simulink model "CTRNN"  (Simulink 7.5)
settings: Solver=ode45  StartTime=0.0  StopTime=10.0  MaxStep=0.1  RelTol=1e-3
settings Model: Creator=richard  LastModifiedBy=richard

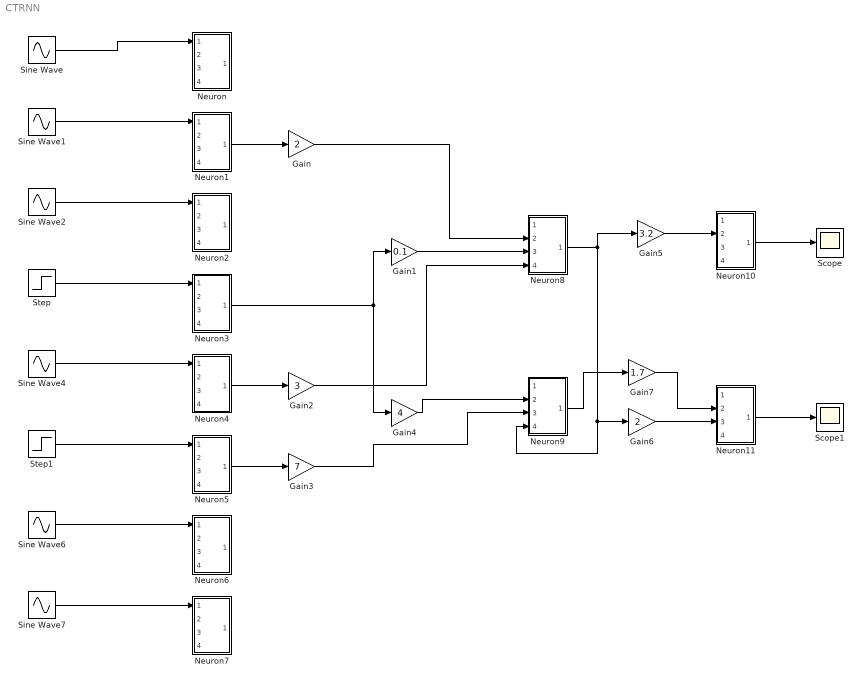
== system CTRNN ==
  Gain : Gain  Gain=2  ParameterDataType=fixdt(1, 16)  ParameterScaling=2^0  OutDataType=fixdt(1, 16)  OutScaling=2^0
  Gain1 : Gain  Gain=0.1  ParameterDataType=fixdt(1, 16)  ParameterScaling=2^0  OutDataType=fixdt(1, 16)  OutScaling=2^0
  Gain2 : Gain  Gain=3  ParameterDataType=fixdt(1, 16)  ParameterScaling=2^0  OutDataType=fixdt(1, 16)  OutScaling=2^0
  Gain3 : Gain  Gain=7  ParameterDataType=fixdt(1, 16)  ParameterScaling=2^0  OutDataType=fixdt(1, 16)  OutScaling=2^0
  Gain4 : Gain  Gain=4  ParameterDataType=fixdt(1, 16)  ParameterScaling=2^0  OutDataType=fixdt(1, 16)  OutScaling=2^0
  Gain5 : Gain  Gain=3.2  ParameterDataType=fixdt(1, 16)  ParameterScaling=2^0  OutDataType=fixdt(1, 16)  OutScaling=2^0
  Gain6 : Gain  Gain=2  ParameterDataType=fixdt(1, 16)  ParameterScaling=2^0  OutDataType=fixdt(1, 16)  OutScaling=2^0
  Gain7 : Gain  Gain=1.7  ParameterDataType=fixdt(1, 16)  ParameterScaling=2^0  OutDataType=fixdt(1, 16)  OutScaling=2^0
  Neuron : Subsystem
  Neuron1 : Subsystem
  Neuron10 : Subsystem
  Neuron11 : Subsystem
  Neuron2 : Subsystem
  Neuron3 : Subsystem
  Neuron4 : Subsystem
  Neuron5 : Subsystem
  Neuron6 : Subsystem
  Neuron7 : Subsystem
  Neuron8 : Subsystem
  Neuron9 : Subsystem
  Scope : Scope
  Scope1 : Scope
  Sine Wave{,1..2,4,6..7} (6 alike) : Sin  Amplitude=1  Bias=0  Frequency=1  Phase=0  Samples=10  SampleTime=0  Offset=0
  Step : Step  SampleTime=0
  Step1 : Step  Time=4  SampleTime=0
  wires:
  Sine Wave7/1 -> Neuron7/1(In1)
  Sine Wave6/1 -> Neuron6/1(In1)
  Step1/1 -> Neuron5/1(In1)
  Sine Wave4/1 -> Neuron4/1(In1)
  Step/1 -> Neuron3/1(In1)
  Sine Wave2/1 -> Neuron2/1(In1)
  Sine Wave1/1 -> Neuron1/1(In1)
  Sine Wave/1 -> Neuron/1(In1)
  Neuron1/1(Out1) -> Gain/1
  Neuron3/1(Out1) -> Gain1/1, Gain4/1
  Neuron4/1(Out1) -> Gain2/1
  Neuron8/1(Out1) -> Neuron9/4(In4), Gain6/1, Gain5/1
  Neuron9/1(Out1) -> Gain7/1
  Neuron10/1(Out1) -> Scope/1
  Neuron11/1(Out1) -> Scope1/1
  Neuron5/1(Out1) -> Gain3/1
  Gain/1 -> Neuron8/2(In2)
  Gain2/1 -> Neuron8/4(In4)
  Gain3/1 -> Neuron9/3(In3)
  Gain1/1 -> Neuron8/3(In3)
  Gain4/1 -> Neuron9/2(In2)
  Gain5/1 -> Neuron10/2(In2)
  Gain6/1 -> Neuron11/3(In3)
  Gain7/1 -> Neuron11/2(In2)

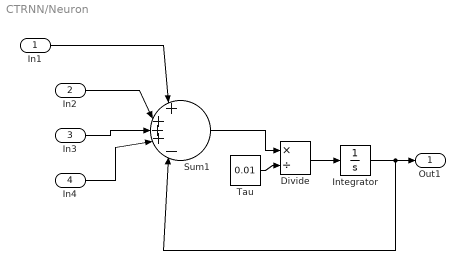
== system CTRNN/Neuron ==
  In1 : Inport
  In2 : Inport  Port=2
  In3 : Inport  Port=3
  In4 : Inport  Port=4  OutDataType=fixdt(1, 16)  OutScaling=2^0
  Divide : Product  Inputs=*/  OutDataType=fixdt(1, 16)  OutScaling=2^-10
  Integrator : Integrator
  Sum1 : Sum  Inputs=|+|+++|-|  OutDataType=fixdt(1, 16)  OutScaling=2^0
  Tau : Constant  Value=0.01  OutDataType=fixdt(1, 16)  OutScaling=2^0
  Out1 : Outport
  wires:
  Sum1/1 -> Divide/1
  Tau/1 -> Divide/2
  Divide/1 -> Integrator/1
  Integrator/1 -> Sum1/5, Out1/1
  In1/1 -> Sum1/1
  In2/1 -> Sum1/2
  In3/1 -> Sum1/3
  In4/1 -> Sum1/4

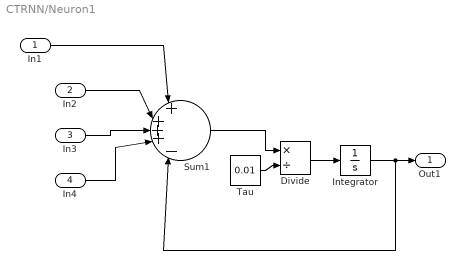
== system CTRNN/Neuron1 ==
  In1 : Inport
  In2 : Inport  Port=2
  In3 : Inport  Port=3
  In4 : Inport  Port=4  OutDataType=fixdt(1, 16)  OutScaling=2^0
  Divide : Product  Inputs=*/  OutDataType=fixdt(1, 16)  OutScaling=2^-10
  Integrator : Integrator
  Sum1 : Sum  Inputs=|+|+++|-|  OutDataType=fixdt(1, 16)  OutScaling=2^0
  Tau : Constant  Value=0.01  OutDataType=fixdt(1, 16)  OutScaling=2^0
  Out1 : Outport
  wires:
  Sum1/1 -> Divide/1
  Tau/1 -> Divide/2
  Divide/1 -> Integrator/1
  Integrator/1 -> Sum1/5, Out1/1
  In1/1 -> Sum1/1
  In2/1 -> Sum1/2
  In3/1 -> Sum1/3
  In4/1 -> Sum1/4

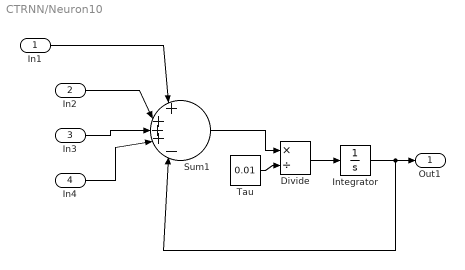
== system CTRNN/Neuron10 ==
  In1 : Inport
  In2 : Inport  Port=2
  In3 : Inport  Port=3
  In4 : Inport  Port=4  OutDataType=fixdt(1, 16)  OutScaling=2^0
  Divide : Product  Inputs=*/  OutDataType=fixdt(1, 16)  OutScaling=2^-10
  Integrator : Integrator
  Sum1 : Sum  Inputs=|+|+++|-|  OutDataType=fixdt(1, 16)  OutScaling=2^0
  Tau : Constant  Value=0.01  OutDataType=fixdt(1, 16)  OutScaling=2^0
  Out1 : Outport
  wires:
  Sum1/1 -> Divide/1
  Tau/1 -> Divide/2
  Divide/1 -> Integrator/1
  Integrator/1 -> Sum1/5, Out1/1
  In1/1 -> Sum1/1
  In2/1 -> Sum1/2
  In3/1 -> Sum1/3
  In4/1 -> Sum1/4

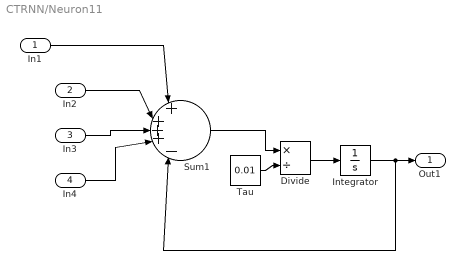
== system CTRNN/Neuron11 ==
  In1 : Inport
  In2 : Inport  Port=2
  In3 : Inport  Port=3
  In4 : Inport  Port=4  OutDataType=fixdt(1, 16)  OutScaling=2^0
  Divide : Product  Inputs=*/  OutDataType=fixdt(1, 16)  OutScaling=2^-10
  Integrator : Integrator
  Sum1 : Sum  Inputs=|+|+++|-|  OutDataType=fixdt(1, 16)  OutScaling=2^0
  Tau : Constant  Value=0.01  OutDataType=fixdt(1, 16)  OutScaling=2^0
  Out1 : Outport
  wires:
  Sum1/1 -> Divide/1
  Tau/1 -> Divide/2
  Divide/1 -> Integrator/1
  Integrator/1 -> Sum1/5, Out1/1
  In1/1 -> Sum1/1
  In2/1 -> Sum1/2
  In3/1 -> Sum1/3
  In4/1 -> Sum1/4

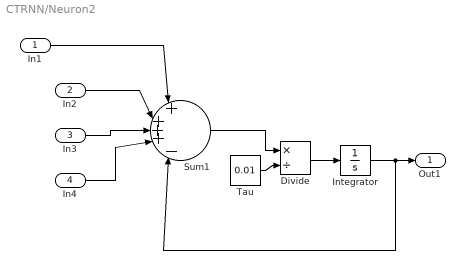
== system CTRNN/Neuron2 ==
  In1 : Inport
  In2 : Inport  Port=2
  In3 : Inport  Port=3
  In4 : Inport  Port=4  OutDataType=fixdt(1, 16)  OutScaling=2^0
  Divide : Product  Inputs=*/  OutDataType=fixdt(1, 16)  OutScaling=2^-10
  Integrator : Integrator
  Sum1 : Sum  Inputs=|+|+++|-|  OutDataType=fixdt(1, 16)  OutScaling=2^0
  Tau : Constant  Value=0.01  OutDataType=fixdt(1, 16)  OutScaling=2^0
  Out1 : Outport
  wires:
  Sum1/1 -> Divide/1
  Tau/1 -> Divide/2
  Divide/1 -> Integrator/1
  Integrator/1 -> Sum1/5, Out1/1
  In1/1 -> Sum1/1
  In2/1 -> Sum1/2
  In3/1 -> Sum1/3
  In4/1 -> Sum1/4

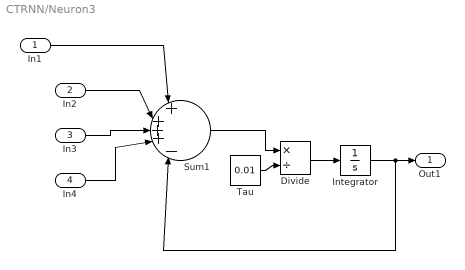
== system CTRNN/Neuron3 ==
  In1 : Inport
  In2 : Inport  Port=2
  In3 : Inport  Port=3
  In4 : Inport  Port=4  OutDataType=fixdt(1, 16)  OutScaling=2^0
  Divide : Product  Inputs=*/  OutDataType=fixdt(1, 16)  OutScaling=2^-10
  Integrator : Integrator
  Sum1 : Sum  Inputs=|+|+++|-|  OutDataType=fixdt(1, 16)  OutScaling=2^0
  Tau : Constant  Value=0.01  OutDataType=fixdt(1, 16)  OutScaling=2^0
  Out1 : Outport
  wires:
  Sum1/1 -> Divide/1
  Tau/1 -> Divide/2
  Divide/1 -> Integrator/1
  Integrator/1 -> Sum1/5, Out1/1
  In1/1 -> Sum1/1
  In2/1 -> Sum1/2
  In3/1 -> Sum1/3
  In4/1 -> Sum1/4

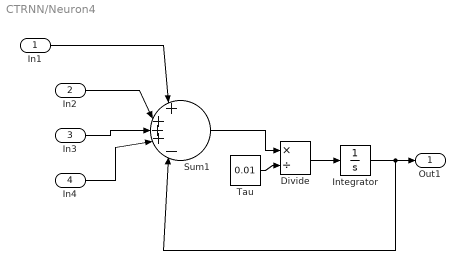
== system CTRNN/Neuron4 ==
  In1 : Inport
  In2 : Inport  Port=2
  In3 : Inport  Port=3
  In4 : Inport  Port=4  OutDataType=fixdt(1, 16)  OutScaling=2^0
  Divide : Product  Inputs=*/  OutDataType=fixdt(1, 16)  OutScaling=2^-10
  Integrator : Integrator
  Sum1 : Sum  Inputs=|+|+++|-|  OutDataType=fixdt(1, 16)  OutScaling=2^0
  Tau : Constant  Value=0.01  OutDataType=fixdt(1, 16)  OutScaling=2^0
  Out1 : Outport
  wires:
  Sum1/1 -> Divide/1
  Tau/1 -> Divide/2
  Divide/1 -> Integrator/1
  Integrator/1 -> Sum1/5, Out1/1
  In1/1 -> Sum1/1
  In2/1 -> Sum1/2
  In3/1 -> Sum1/3
  In4/1 -> Sum1/4

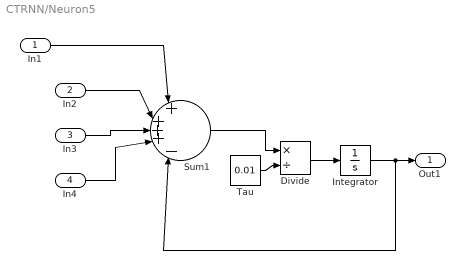
== system CTRNN/Neuron5 ==
  In1 : Inport
  In2 : Inport  Port=2
  In3 : Inport  Port=3
  In4 : Inport  Port=4  OutDataType=fixdt(1, 16)  OutScaling=2^0
  Divide : Product  Inputs=*/  OutDataType=fixdt(1, 16)  OutScaling=2^-10
  Integrator : Integrator
  Sum1 : Sum  Inputs=|+|+++|-|  OutDataType=fixdt(1, 16)  OutScaling=2^0
  Tau : Constant  Value=0.01  OutDataType=fixdt(1, 16)  OutScaling=2^0
  Out1 : Outport
  wires:
  Sum1/1 -> Divide/1
  Tau/1 -> Divide/2
  Divide/1 -> Integrator/1
  Integrator/1 -> Sum1/5, Out1/1
  In1/1 -> Sum1/1
  In2/1 -> Sum1/2
  In3/1 -> Sum1/3
  In4/1 -> Sum1/4

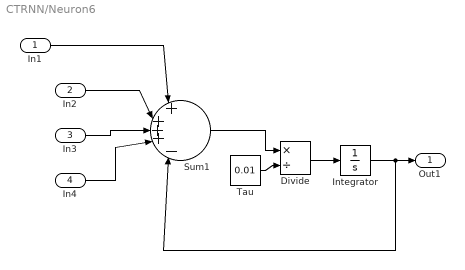
== system CTRNN/Neuron6 ==
  In1 : Inport
  In2 : Inport  Port=2
  In3 : Inport  Port=3
  In4 : Inport  Port=4  OutDataType=fixdt(1, 16)  OutScaling=2^0
  Divide : Product  Inputs=*/  OutDataType=fixdt(1, 16)  OutScaling=2^-10
  Integrator : Integrator
  Sum1 : Sum  Inputs=|+|+++|-|  OutDataType=fixdt(1, 16)  OutScaling=2^0
  Tau : Constant  Value=0.01  OutDataType=fixdt(1, 16)  OutScaling=2^0
  Out1 : Outport
  wires:
  Sum1/1 -> Divide/1
  Tau/1 -> Divide/2
  Divide/1 -> Integrator/1
  Integrator/1 -> Sum1/5, Out1/1
  In1/1 -> Sum1/1
  In2/1 -> Sum1/2
  In3/1 -> Sum1/3
  In4/1 -> Sum1/4

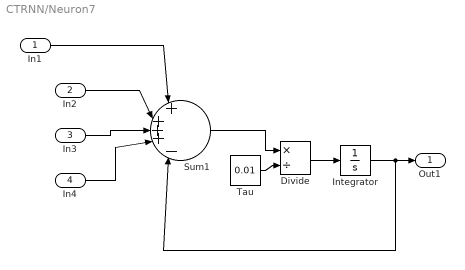
== system CTRNN/Neuron7 ==
  In1 : Inport
  In2 : Inport  Port=2
  In3 : Inport  Port=3
  In4 : Inport  Port=4  OutDataType=fixdt(1, 16)  OutScaling=2^0
  Divide : Product  Inputs=*/  OutDataType=fixdt(1, 16)  OutScaling=2^-10
  Integrator : Integrator
  Sum1 : Sum  Inputs=|+|+++|-|  OutDataType=fixdt(1, 16)  OutScaling=2^0
  Tau : Constant  Value=0.01  OutDataType=fixdt(1, 16)  OutScaling=2^0
  Out1 : Outport
  wires:
  Sum1/1 -> Divide/1
  Tau/1 -> Divide/2
  Divide/1 -> Integrator/1
  Integrator/1 -> Sum1/5, Out1/1
  In1/1 -> Sum1/1
  In2/1 -> Sum1/2
  In3/1 -> Sum1/3
  In4/1 -> Sum1/4

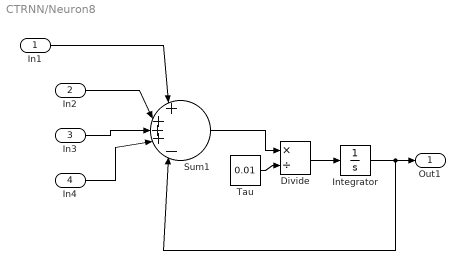
== system CTRNN/Neuron8 ==
  In1 : Inport
  In2 : Inport  Port=2
  In3 : Inport  Port=3
  In4 : Inport  Port=4  OutDataType=fixdt(1, 16)  OutScaling=2^0
  Divide : Product  Inputs=*/  OutDataType=fixdt(1, 16)  OutScaling=2^-10
  Integrator : Integrator
  Sum1 : Sum  Inputs=|+|+++|-|  OutDataType=fixdt(1, 16)  OutScaling=2^0
  Tau : Constant  Value=0.01  OutDataType=fixdt(1, 16)  OutScaling=2^0
  Out1 : Outport
  wires:
  Sum1/1 -> Divide/1
  Tau/1 -> Divide/2
  Divide/1 -> Integrator/1
  Integrator/1 -> Sum1/5, Out1/1
  In1/1 -> Sum1/1
  In2/1 -> Sum1/2
  In3/1 -> Sum1/3
  In4/1 -> Sum1/4

== system CTRNN/Neuron9 ==
  In1 : Inport
  In2 : Inport  Port=2
  In3 : Inport  Port=3
  In4 : Inport  Port=4  OutDataType=fixdt(1, 16)  OutScaling=2^0
  Divide : Product  Inputs=*/  OutDataType=fixdt(1, 16)  OutScaling=2^-10
  Integrator : Integrator
  Sum1 : Sum  Inputs=|+|+++|-|  OutDataType=fixdt(1, 16)  OutScaling=2^0
  Tau : Constant  Value=0.01  OutDataType=fixdt(1, 16)  OutScaling=2^0
  Out1 : Outport
  wires:
  Sum1/1 -> Divide/1
  Tau/1 -> Divide/2
  Divide/1 -> Integrator/1
  Integrator/1 -> Sum1/5, Out1/1
  In1/1 -> Sum1/1
  In2/1 -> Sum1/2
  In3/1 -> Sum1/3
  In4/1 -> Sum1/4
